simulink model "SMC_Leukemia_nonmono"  (R2024b)
settings: Solver=VariableStepAuto  StartTime=0.0  StopTime=30  RelTol=1e-3  EnableMultiTasking=on
undefined symbols (not defined in the file or in its folder): DiscIntNeverNeededParam
settings Model: Creator=engry  LastModifiedBy=munir
settings SolverCC: DateTimeAtSimulationTimeZero=[]  AlgebraicLoopSolver=TrustRegion
settings DataIOCC: ReturnWorkspaceOutputs=off
settings OptimizationCC: LifeSpan=inf
settings DebuggingCC: UnconnectedInputMsg=warning  UnconnectedOutputMsg=warning  UnconnectedLineMsg=warning  SFUnexpectedBacktrackingDiag=warning  SFNoUnconditionalDefaultTransitionDiag=warning  ArithmeticOperatorsInVariantConditions=warning
settings ModelReferenceCC: EnableRefExpFcnMdlSchedulingChecks=on
settings SFSimCC: SimUseLocalCustomCode=off  CustomCodeUndefinedFunction=UseInterfaceOnly
settings RTWCC: RTWUseLocalCustomCode=off  GPUComputeCapability=3.5
settings CodeAppCC: StateflowObjectComments=on
settings GRTTargetCC: TargetLangStandard=C89/C90 (ANSI)
settings ConfigComp: CovMetricSettings=dw  CovSaveCumulativeToWorkspaceVar=on  CovSaveSingleToWorkspaceVar=on  CovExternalEMLEnable=off

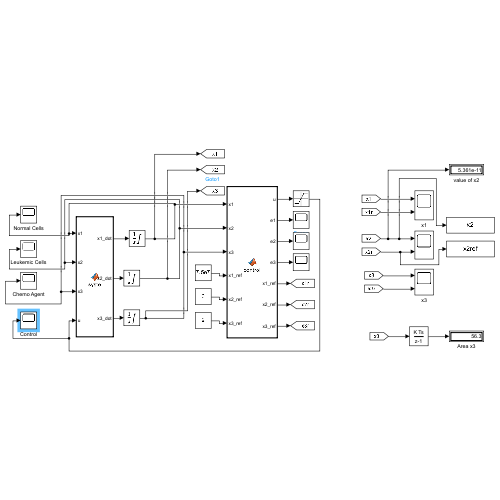
[thumbnail: Simulink's stored preview of the top-level diagram]
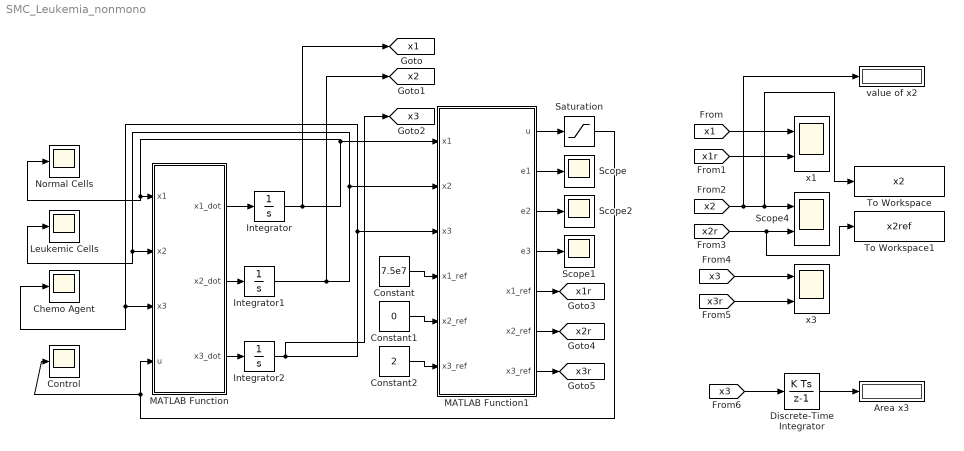
== system SMC_Leukemia_nonmono ==
  Area x3 : Display
  Chemo Agent : Scope
  Constant : Constant  Value=7.5e7
  Constant1 : Constant  Value=0
  Constant2 : Constant  Value=2
  Control : Scope
  Discrete-Time Integrator : DiscreteIntegrator  SampleTime=-1  ICPrevOutput=DiscIntNeverNeededParam  ICPrevScaledInput=DiscIntNeverNeededParam
  Integrator : Integrator  InitialCondition=1e8  LimitOutput=on  LowerSaturationLimit=7.5e7
  Integrator1 : Integrator  InitialCondition=1.8e8  LimitOutput=on  LowerSaturationLimit=0
  Integrator2 : Integrator  LimitOutput=on  UpperSaturationLimit=2  LowerSaturationLimit=0
  Leukemic Cells : Scope
  MATLAB Function : MATLAB Function  TreatAsAtomicUnit=on
  MATLAB Function1 : MATLAB Function  TreatAsAtomicUnit=on
  Normal Cells : Scope
  Saturation : Saturate  UpperLimit=1  LowerLimit=0  ZeroCross=off  RndMeth=Ceiling
  Scope : Scope
  Scope1 : Scope
  Scope2 : Scope
  Scope4 : Scope  NumInputPorts=2
  To Workspace : ToWorkspace  VariableName=x2  SampleTime=-1
      settings: Save2DSignal=2-D array (concatenate along first dimension)
  To Workspace1 : ToWorkspace  VariableName=x2ref  SampleTime=-1
      settings: Save2DSignal=2-D array (concatenate along first dimension)
  value of x2 : Display
  x1 : Scope  NumInputPorts=2
  x3 : Scope  NumInputPorts=2
  tag scope: x1=global, x1r=global, x2=global, x2r=global, x3=global, x3r=global
  wires:
  MATLAB Function/2(x2_dot) -> Integrator1/1
  MATLAB Function/3(x3_dot) -> Integrator2/1
  Integrator/1 -> Normal Cells/1, MATLAB Function/1(x1), MATLAB Function1/1(x1), [x1]
  Integrator2/1 -> [x3], Chemo Agent/1, MATLAB Function/3(x3), MATLAB Function1/3(x3)
  Constant/1 -> MATLAB Function1/4("x1_ref ")
  Constant1/1 -> MATLAB Function1/5("x2_ref ")
  Constant2/1 -> MATLAB Function1/6("x3_ref ")
  MATLAB Function1/1(u) -> Saturation/1
  Saturation/1 -> Control/1, MATLAB Function/4(u)
  MATLAB Function1/2(e1) -> Scope/1
  MATLAB Function1/3(e2) -> Scope2/1
  MATLAB Function1/4(e3) -> Scope1/1
  Integrator1/1 -> [x2], MATLAB Function/2(x2), Leukemic Cells/1, MATLAB Function1/2(x2)
  MATLAB Function/1(x1_dot) -> Integrator/1
  [x3r] -> x3/2
  [x1] -> x1/1
  [x2r] -> To Workspace1/1, Scope4/2
  [x3] -> x3/1
  [x1r] -> x1/2
  [x2] -> value of x2/1, To Workspace/1, Scope4/1
  MATLAB Function1/5(x1_ref) -> [x1r]
  MATLAB Function1/6(x2_ref) -> [x2r]
  MATLAB Function1/7(x3_ref) -> [x3r]
  [x3] -> Discrete-Time Integrator/1
  Discrete-Time Integrator/1 -> Area x3/1

== matlab function SMC_Leukemia_nonmono/MATLAB Function1 ==
  data: u output; e1 output; e2 output; e3 output; x1 input; x2 input; x3 input; x1_ref input; x2_ref input; x3_ref input; x1_ref output; x2_ref output; x3_ref output
function [u,e1,e2,e3,x1_ref,x2_ref,x3_ref]=control(x1,x2,x3,x1_ref,x2_ref,x3_ref)

r_l = 0.1;
r_n = 0.1;
lambda_l = 2.5;
lambda_n = 1.4;
La = 1e10;
Na = 1e10;
d = 0.4;
m1 = 0.04; %gamma_n
m2 = 0.04; %%gamma_l
c = 1e-1;
b1=0.01;
b2=0.01;

x1_dot = r_n * x1 *log(Na) - r_n*x1*real(log(complex(x1))) - m1*x1 - (c*x1*x2)/(1+x2)-lambda_n*x1*(x3 - b1*x3^2);

x2_dot = r_l*x2 *log(La) - r_l*x2*real(log(complex(x2))) - m2*x2 - lambda_l*x2*(x3-b2*x3^2);



a1=1e-15;
a2=1e-15;
a3=0.1;
alpha=0.95;
phi=0.75;
k=1;

e1=x1-x1_ref;
e2=x2-x2_ref;
e3=x3-x3_ref;

s=a1*e1+a2*e2+a3*e3;

u=(-k*((abs(s))^alpha)*(sign(s/phi))/a3) - (a1*x1_dot/a3) - (a2*x2_dot/a3) + (d*x3);

== matlab function SMC_Leukemia_nonmono/MATLAB Function ==
  data: x1 input; x1_dot output; x2 input; x3 input; x2_dot output; x3_dot output; u input
function[x1_dot, x2_dot, x3_dot] = syste(x1, x2, x3, u)

r_l = 0.1;
r_n = 0.1;
lambda_l = 2.5;
lambda_n = 1.4;
La = 1e10;
Na = 1e10;
d = 0.4;
m1 = 0.04;
m2 = 0.04;
c = 1e-1;
b1=0.01;
b2=0.01;

%System Model
x1_dot = r_n * x1 *log(Na) - r_n*x1*real(log(complex(x1))) - m1*x1 - (c*x1*x2)/(1+x2)-lambda_n*x1*(x3 - b1*x3^2);

x2_dot = r_l*x2 *log(La) - r_l*x2*real(log(complex(x2))) - m2*x2 - lambda_l*x2*(x3-b2*x3^2);

x3_dot = -d*x3 + u;
